simulink model "control_law_testing"  (R2023a)
settings: Solver=VariableStepAuto  StartTime=0.0  StopTime=20  RelTol=1e-6
libraries: aerolibutil x4, matrix_library x2, dspinverses x1, sharedutil x1
settings Model: Creator=owenw  LastModifiedBy=owenw

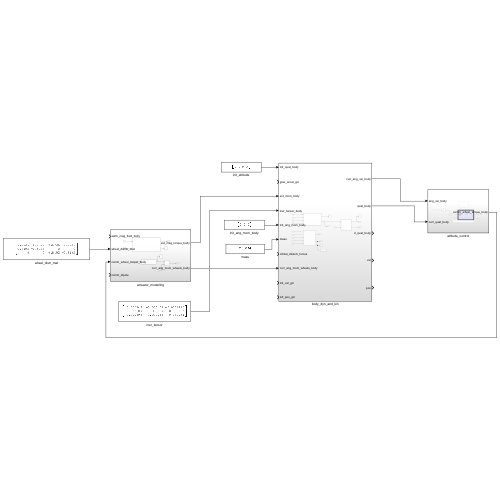
[thumbnail: Simulink's stored preview of the top-level diagram]
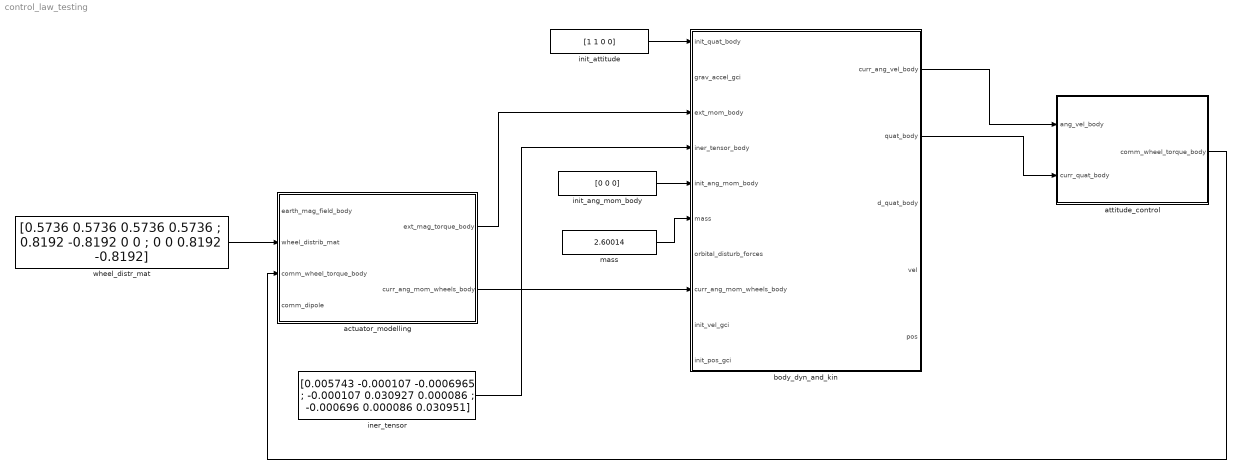
== system control_law_testing ==
  actuator_modelling : Subsystem
  attitude_control : Subsystem
  body_dyn_and_kin : Subsystem
  iner_tensor : Constant  Value=[0.005743 -0.000107 -0.0006965 ; -0.000107 0.030927 0.000086 ; -0.000696 0.000086 0.030951]
  init_ang_mom_body : Constant  Value=[0 0 0]
  init_attitude : Constant  Value=[1 1 0 0]
  mass : Constant  Value=2.60014
  wheel_distr_mat : Constant  Value=[0.5736 0.5736 0.5736 0.5736 ; 0.8192 -0.8192 0 0 ; 0 0 0.8192 -0.8192]
  wires:
  actuator_modelling/2(curr_ang_mom_wheels_body) -> body_dyn_and_kin/8(curr_ang_mom_wheels_body)
  attitude_control/1(comm_wheel_torque_body) -> actuator_modelling/3(comm_wheel_torque_body)
  wheel_distr_mat/1 -> actuator_modelling/2(wheel_distrib_mat)
  iner_tensor/1 -> body_dyn_and_kin/4(iner_tensor_body)
  init_ang_mom_body/1 -> body_dyn_and_kin/5(init_ang_mom_body)
  body_dyn_and_kin/1(curr_ang_vel_body) -> attitude_control/1(ang_vel_body)
  body_dyn_and_kin/2(quat_body) -> attitude_control/2(curr_quat_body)
  mass/1 -> body_dyn_and_kin/6(mass)
  actuator_modelling/1(ext_mag_torque_body) -> body_dyn_and_kin/3(ext_mom_body)
  init_attitude/1 -> body_dyn_and_kin/1(init_quat_body)

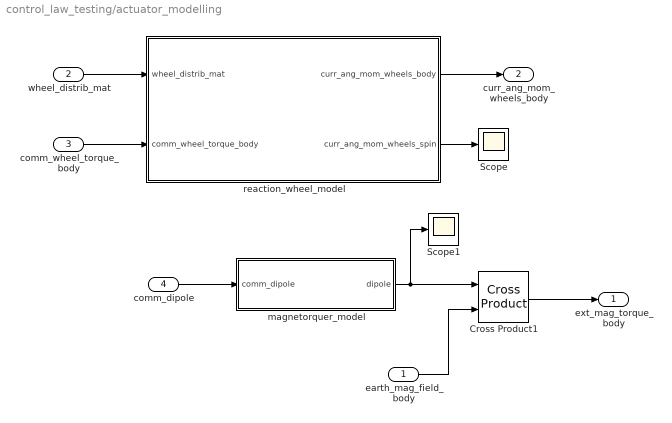
== system control_law_testing/actuator_modelling ==
  earth_mag_field_body : Inport
  wheel_distrib_mat : Inport  Port=2
  comm_wheel_torque_body : Inport  Port=3
  comm_dipole : Inport  Port=4
  Cross Product1 : matrix_library/Cross Product
  Scope : Scope
  Scope1 : Scope
  magnetorquer_model : Subsystem
  reaction_wheel_model : Subsystem
  ext_mag_torque_body : Outport
  curr_ang_mom_wheels_body : Outport  Port=2
  wires:
  reaction_wheel_model/2(curr_ang_mom_wheels_spin) -> Scope/1
  magnetorquer_model/1(dipole) -> Scope1/1, Cross Product1/1
  Cross Product1/1 -> ext_mag_torque_body/1
  wheel_distrib_mat/1 -> reaction_wheel_model/1(wheel_distrib_mat)
  comm_wheel_torque_body/1 -> reaction_wheel_model/2(comm_wheel_torque_body)
  earth_mag_field_body/1 -> Cross Product1/2
  comm_dipole/1 -> magnetorquer_model/1(comm_dipole)
  reaction_wheel_model/1(curr_ang_mom_wheels_body) -> curr_ang_mom_wheels_body/1

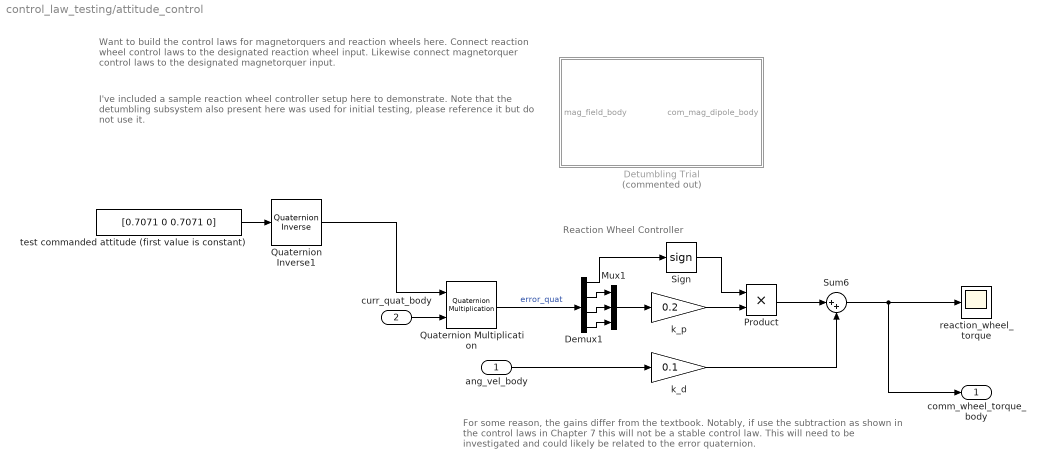
== system control_law_testing/attitude_control ==
  note: For some reason, the gains differ from the textbook. Notably, if use the subtraction as shown in the control laws in Chapter 7 this will not be a stable control law. This will need to be investigated and could likely be related to the error quaternion.
  note: Reaction Wheel Controller
  note: I've included a sample reaction wheel controller setup here to demonstrate. Note that the detumbling subsystem also present here was used for initial testing, please reference it but do not use it.
  note: Want to build the control laws for magnetorquers and reaction wheels here. Connect reaction wheel control laws to the designated reaction wheel input. Likewise connect magnetorquer control laws to the designated magnetorquer input.
  ang_vel_body : Inport
  curr_quat_body : Inport  Port=2
  Demux1 : Demux
  Detumbling Trial : Subsystem  Commented=on
  Mux1 : Mux  Inputs=3
  Product : Product
  Quaternion Inverse1 : aerolibutil/Quaternion Inverse
  Quaternion Multiplication : aerolibutil/Quaternion Multiplication
  Sign : Signum
  Sum6 : Sum  Inputs=|++
  k_d : Gain  Gain=0.1
  k_p : Gain  Gain=0.2
  reaction_wheel_torque : Scope
  test commanded attitude (first value is constant) : Constant  Value=[0.7071 0 0.7071 0]
  comm_wheel_torque_body : Outport
  wires:
  Quaternion Multiplication/1 -> Demux1/1  "error_quat"
  curr_quat_body/1 -> Quaternion Multiplication/2
  ang_vel_body/1 -> k_d/1
  Quaternion Inverse1/1 -> Quaternion Multiplication/1
  Sum6/1 -> comm_wheel_torque_body/1, reaction_wheel_torque/1
  Demux1/3 -> Mux1/2
  Demux1/2 -> Mux1/1
  Demux1/4 -> Mux1/3
  k_p/1 -> Product/2
  Demux1/1 -> Sign/1
  Mux1/1 -> k_p/1
  Sign/1 -> Product/1
  Product/1 -> Sum6/1
  k_d/1 -> Sum6/2
  test commanded attitude (first value is constant)/1 -> Quaternion Inverse1/1

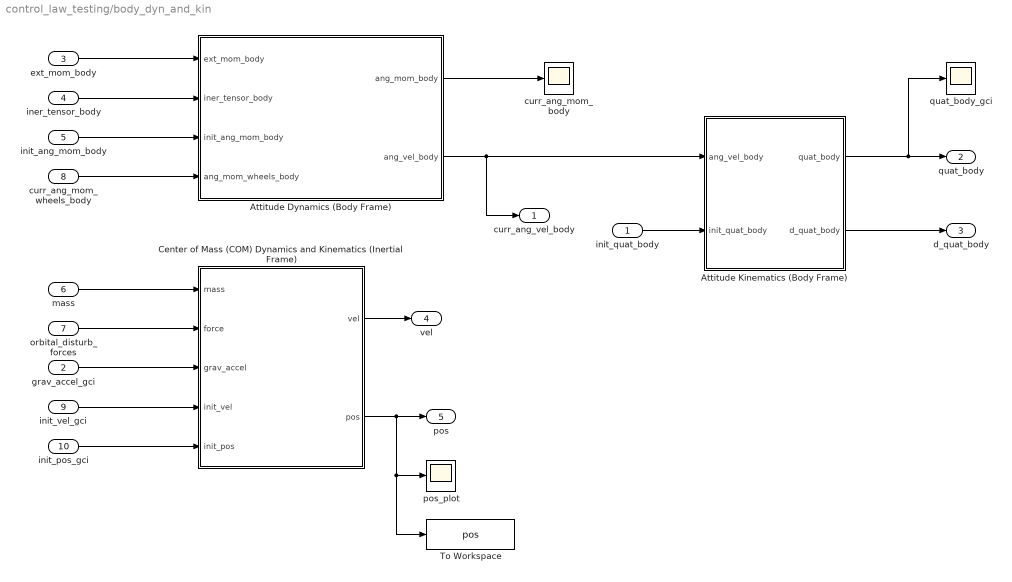
== system control_law_testing/body_dyn_and_kin ==
  init_quat_body : Inport
  grav_accel_gci : Inport  Port=2
  ext_mom_body : Inport  Port=3
  iner_tensor_body : Inport  Port=4
  init_ang_mom_body : Inport  Port=5
  mass : Inport  Port=6
  orbital_disturb_forces : Inport  Port=7
  curr_ang_mom_wheels_body : Inport  Port=8
  init_vel_gci : Inport  Port=9
  init_pos_gci : Inport  Port=10
  Attitude Dynamics (Body Frame) : Subsystem
  Attitude Kinematics (Body Frame) : Subsystem
  Center of Mass (COM) Dynamics and Kinematics (Inertial Frame) : Subsystem
  To Workspace : ToWorkspace  VariableName=pos  SampleTime=-1
  curr_ang_mom_body : Scope
  pos_plot : Scope
  quat_body_gci : Scope
  curr_ang_vel_body : Outport
  quat_body : Outport  Port=2
  d_quat_body : Outport  Port=3
  vel : Outport  Port=4
  pos : Outport  Port=5
  wires:
  init_quat_body/1 -> Attitude Kinematics (Body Frame)/2(init_quat_body)
  grav_accel_gci/1 -> Center of Mass (COM) Dynamics and Kinematics (Inertial Frame)/3(grav_accel)
  ext_mom_body/1 -> Attitude Dynamics (Body Frame)/1(ext_mom_body)
  Attitude Dynamics (Body Frame)/2(ang_vel_body) -> Attitude Kinematics (Body Frame)/1(ang_vel_body), curr_ang_vel_body/1
  iner_tensor_body/1 -> Attitude Dynamics (Body Frame)/2(iner_tensor_body)
  init_vel_gci/1 -> Center of Mass (COM) Dynamics and Kinematics (Inertial Frame)/4(init_vel)
  orbital_disturb_forces/1 -> Center of Mass (COM) Dynamics and Kinematics (Inertial Frame)/2(force)
  curr_ang_mom_wheels_body/1 -> Attitude Dynamics (Body Frame)/4(ang_mom_wheels_body)
  init_pos_gci/1 -> Center of Mass (COM) Dynamics and Kinematics (Inertial Frame)/5(init_pos)
  Center of Mass (COM) Dynamics and Kinematics (Inertial Frame)/2(pos) -> To Workspace/1, pos_plot/1, pos/1
  Attitude Kinematics (Body Frame)/2(d_quat_body) -> d_quat_body/1
  Attitude Kinematics (Body Frame)/1(quat_body) -> quat_body_gci/1, quat_body/1
  mass/1 -> Center of Mass (COM) Dynamics and Kinematics (Inertial Frame)/1(mass)
  init_ang_mom_body/1 -> Attitude Dynamics (Body Frame)/3(init_ang_mom_body)
  Attitude Dynamics (Body Frame)/1(ang_mom_body) -> curr_ang_mom_body/1
  Center of Mass (COM) Dynamics and Kinematics (Inertial Frame)/1(vel) -> vel/1

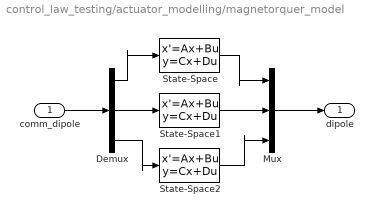
== system control_law_testing/actuator_modelling/magnetorquer_model ==
  comm_dipole : Inport
  Demux : Demux  Outputs=3
  Mux : Mux  Inputs=3
  State-Space : StateSpace  A=-71.31  B=8  C=8.914  D=0  InitialCondition=0
  State-Space1 : StateSpace  A=-71.31  B=8  C=8.914  D=0  InitialCondition=0
  State-Space2 : StateSpace  A=-71.31  B=8  C=8.914  D=0  InitialCondition=0
  dipole : Outport
  wires:
  State-Space/1 -> Mux/1
  State-Space2/1 -> Mux/3
  State-Space1/1 -> Mux/2
  Demux/2 -> State-Space1/1
  Demux/1 -> State-Space/1
  Demux/3 -> State-Space2/1
  Mux/1 -> dipole/1
  comm_dipole/1 -> Demux/1

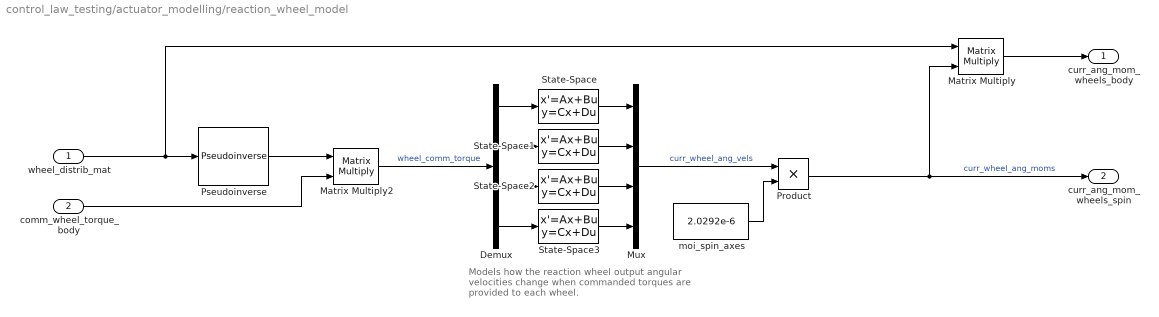
== system control_law_testing/actuator_modelling/reaction_wheel_model ==
  note: Models how the reaction wheel output angular velocities change when commanded torques are provided to each wheel.
  wheel_distrib_mat : Inport
  comm_wheel_torque_body : Inport  Port=2
  Demux : Demux
  Matrix Multiply : Product  Multiplication=Matrix(*)
  Matrix Multiply2 : Product  Multiplication=Matrix(*)
  Mux : Mux
  Product : Product
  Pseudoinverse : dspinverses/Pseudoinverse  wanterr=off  SimulateUsing=Interpreted execution
  State-Space{,1..3} (4 alike) : StateSpace  A=-0.02216  B=512  C=962.5  D=0  InitialCondition=0  ParameterTunability=Unconstrained
  moi_spin_axes : Constant  Value=2.0292e-6
  curr_ang_mom_wheels_body : Outport
  curr_ang_mom_wheels_spin : Outport  Port=2
  wires:
  Demux/1 -> State-Space/1
  Demux/2 -> State-Space1/1
  Demux/4 -> State-Space3/1
  State-Space/1 -> Mux/1
  Pseudoinverse/1 -> Matrix Multiply2/1
  wheel_distrib_mat/1 -> Matrix Multiply/1, Pseudoinverse/1
  State-Space1/1 -> Mux/2
  moi_spin_axes/1 -> Product/2
  Mux/1 -> Product/1  "curr_wheel_ang_vels"
  Product/1 -> curr_ang_mom_wheels_spin/1, Matrix Multiply/2  "curr_wheel_ang_moms"
  Matrix Multiply2/1 -> Demux/1  "wheel_comm_torque"
  State-Space3/1 -> Mux/4
  State-Space2/1 -> Mux/3
  Demux/3 -> State-Space2/1
  comm_wheel_torque_body/1 -> Matrix Multiply2/2
  Matrix Multiply/1 -> curr_ang_mom_wheels_body/1

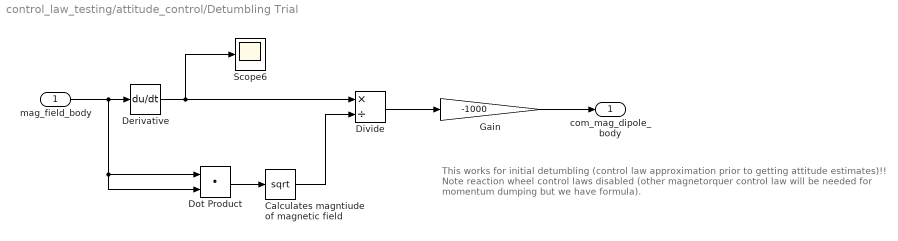
== system control_law_testing/attitude_control/Detumbling Trial ==
  note: This works for initial detumbling (control law approximation prior to getting attitude estimates)!! Note reaction wheel control laws disabled (other magnetorquer control law will be needed for momentum dumping but we have formula).
  mag_field_body : Inport
  Calculates magntiude of magnetic field : Sqrt
  Derivative : Derivative
  Divide : Product  Inputs=*/
  Dot Product : DotProduct  OutDataTypeStr=Inherit: Inherit via internal rule
  Gain : Gain  Gain=-1000
  Scope6 : Scope
  com_mag_dipole_body : Outport
  wires:
  Calculates magntiude of magnetic field/1 -> Divide/2
  Gain/1 -> com_mag_dipole_body/1
  Dot Product/1 -> Calculates magntiude of magnetic field/1
  Divide/1 -> Gain/1
  mag_field_body/1 -> Derivative/1, Dot Product/2, Dot Product/1
  Derivative/1 -> Divide/1, Scope6/1

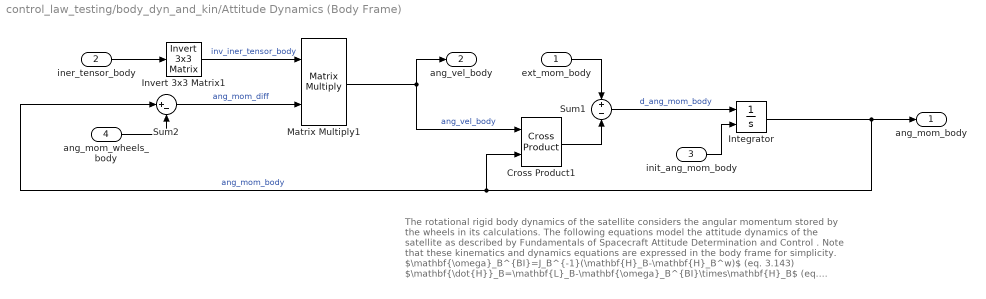
== system control_law_testing/body_dyn_and_kin/Attitude Dynamics (Body Frame) ==
  note: The rotational rigid body dynamics of the satellite considers the angular momentum stored by the wheels in its calculations. The following equations model the attitude dynamics of the satellite as described by Fundamentals of Spacecraft Attitude Determination and Control . Note that these kinematics and dynamics equations are expressed in the body frame for simplicity.
      |
      | $\mathbf{\omega}_B^{BI}=J_B^{-1}(\mathbf{H}_B-\mathbf{H}_B^w)$ (eq. 3.143)
      | $\mathbf{\dot{H}}_B=\mathbf{L}_B-\mathbf{\omega}_B^{BI}\times\mathbf{H}_B$ (eq. 3.80)
      |
      | $\mathbf{\omega}_B^{BI}$ - angular velocity of satellite in body frame
      | $J_B$ - inertia tensor of satellite in body frame
      | $\mathbf{H}_B$ - total angular momentum of satellite in body frame
      | $\mathbf{H}_B^w$ - total angular momentum of wheels in body frame
      | $\mathbf{L}_B$ - moment applied to spacecraft in the body frame
  ext_mom_body : Inport
  iner_tensor_body : Inport  Port=2
  init_ang_mom_body : Inport  Port=3
  ang_mom_wheels_body : Inport  Port=4
  Cross Product1 : matrix_library/Cross Product
  Integrator : Integrator  InitialConditionSource=external
  Invert 3x3 Matrix1 : aerolibutil/Invert  3x3 Matrix
  Matrix Multiply1 : Product  Multiplication=Matrix(*)
  Sum1 : Sum  Inputs=+-
  Sum2 : Sum  Inputs=|+-
  ang_mom_body : Outport
  ang_vel_body : Outport  Port=2
  wires:
  Invert 3x3 Matrix1/1 -> Matrix Multiply1/1  "inv_iner_tensor_body"
  iner_tensor_body/1 -> Invert 3x3 Matrix1/1
  ang_mom_wheels_body/1 -> Sum2/2
  Integrator/1 -> ang_mom_body/1, Sum2/1, Cross Product1/2  "ang_mom_body"
  init_ang_mom_body/1 -> Integrator/2
  Matrix Multiply1/1 -> Cross Product1/1, ang_vel_body/1  "ang_vel_body"
  Sum2/1 -> Matrix Multiply1/2  "ang_mom_diff"
  Sum1/1 -> Integrator/1  "d_ang_mom_body"
  ext_mom_body/1 -> Sum1/1
  Cross Product1/1 -> Sum1/2

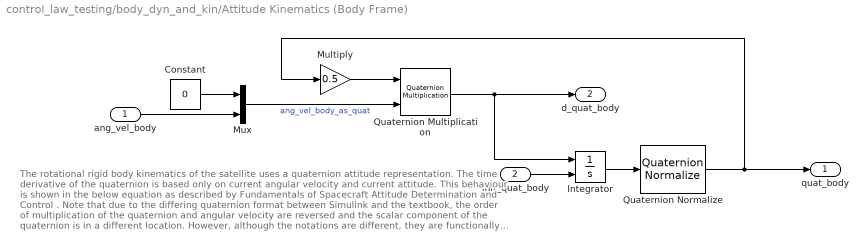
== system control_law_testing/body_dyn_and_kin/Attitude Kinematics (Body Frame) ==
  note: The rotational rigid body kinematics of the satellite uses a quaternion attitude representation. The time derivative of the quaternion is based only on current angular velocity and current attitude. This behaviour is shown in the below equation as described by Fundamentals of Spacecraft Attitude Determination and Control . Note that due to the differing quaternion format between Simulink and the textbook, the order of multiplication of the quaternion and angular velocity are reversed and the scalar component of the quaternion is in a different location. However, although the notations are different, they are functionally the same.
      |
      | $\mathbf{\dot{q}}_{BI}=\frac{1}{2}\mathbf{q}_{BI}\cdot\mathbf{\omega}_B^{BI}=\frac{1}{2}\mathbf{q}_{BI}\cdot\left[\matrix{0 \cr \mathbf{\omega}_B^{BI}}\right]$ (eq. 3.79d)
      |
      | Note that in the above equation, multiplication between a quaternion and vector requires transforming the vector to a quaternion with scalar component of 0, as seen on the RHS.
      |
      | $\mathbf{q}_{BI}$ - current attitude of the spacecraft (rotation from inertial frame to body frame as specified in the inertial frame)
      | $\mathbf{\omega}_{B}^{BI}$ - angular velocity of satellite in body frame
  ang_vel_body : Inport
  init_quat_body : Inport  Port=2
  Constant : Constant  Value=0
  Integrator : Integrator  InitialConditionSource=external
  Multiply : Gain  Gain=0.5
  Mux : Mux  Inputs=2
  Quaternion Multiplication : aerolibutil/Quaternion Multiplication
  Quaternion Normalize : sharedutil/Quaternion Normalize  aMode=aMode
  quat_body : Outport
  d_quat_body : Outport  Port=2
  wires:
  Constant/1 -> Mux/1
  ang_vel_body/1 -> Mux/2
  Multiply/1 -> Quaternion Multiplication/1
  init_quat_body/1 -> Integrator/2
  Quaternion Multiplication/1 -> d_quat_body/1, Integrator/1
  Mux/1 -> Quaternion Multiplication/2  "ang_vel_body_as_quat"
  Integrator/1 -> Quaternion Normalize/1
  Quaternion Normalize/1 -> Multiply/1, quat_body/1

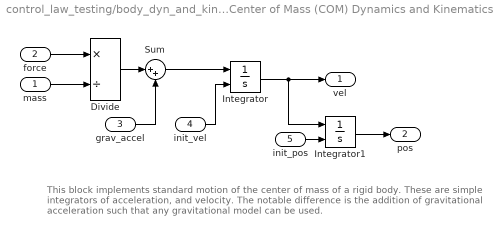
== system control_law_testing/body_dyn_and_kin/Center of Mass (COM) Dynamics and Kinematics (Inertial Frame) ==
  note: This block implements standard motion of the center of mass of a rigid body. These are simple integrators of acceleration, and velocity. The notable difference is the addition of gravitational acceleration such that any gravitational model can be used.
  mass : Inport
  force : Inport  Port=2
  grav_accel : Inport  Port=3
  init_vel : Inport  Port=4
  init_pos : Inport  Port=5
  Divide : Product  Inputs=*/
  Integrator : Integrator  InitialConditionSource=external
  Integrator1 : Integrator  InitialConditionSource=external
  Sum : Sum  Inputs=|++
  vel : Outport
  pos : Outport  Port=2
  wires:
  init_vel/1 -> Integrator/2
  init_pos/1 -> Integrator1/2
  Divide/1 -> Sum/1
  grav_accel/1 -> Sum/2
  mass/1 -> Divide/2
  force/1 -> Divide/1
  Integrator/1 -> vel/1, Integrator1/1
  Integrator1/1 -> pos/1
  Sum/1 -> Integrator/1
